simulink model "Simulink_serial_example"  (Simulink 10.0)
settings: Solver=FixedStepDiscrete  StartTime=0.0  StopTime=1056  RelTol=1e-3  EnableMultiTasking=on
undefined symbols (not defined in the file): D, fdesignblkfcn, gcbh
libraries: dspsigops x42, instrumentlib x1, dspsigattribs x1
settings Model: Creator=skolak  LastModifiedBy=bhisma
settings DataIOCC: LimitDataPoints=on  SignalLoggingSaveFormat=ModelDataLogs
settings OptimizationCC: InitFltsAndDblsToZero=on
settings DebuggingCC: SaveWithParameterizedLinksMsg=none  SignalResolutionControl=TryResolveAllWithWarning  SolverPrmCheckMsg=warning  MultiTaskDSMMsg=warning  MultiTaskCondExecSysMsg=none  FcnCallInpInsideContextMsg=warning
settings SFSimCC: SimUseLocalCustomCode=on  CustomCodeUndefinedFunction=FilterOut
settings RTWCC: RTWUseLocalCustomCode=on
settings GRTTargetCC: TargetFcnLib=ansi_tfl_tmw.mat

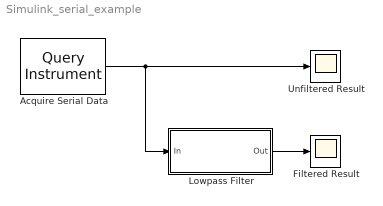
== system Simulink_serial_example ==
  Acquire Serial Data : instrumentlib/Query Instrument  sampleTime=1  isWorkspaceObject=off  timeout=10  inputBufferSize=10000  protocol=Serial  serialPort=COM1  baudRate=9600  gpibVendor=Advantech  boardIndex=0  primaryAddress=1  secondaryAddress=0  visaVendor=Agilent  visaSerialPort=0  chassisIndex=0  logicalAddress=0  tcpRemoteHost='127.0.0.1'  tcpRemotePort=4500  udpRemoteHost='127.0.0.1'  udpRemotePort=9090  visaTCPBoardIndex=0  visaTCPRemoteHost='127.0.0.1'  usbBoardIndex=0  usbManufID=0  usbModelCode=0  usbSerialNumber=0  initAction=Send ASCII Commands  initCommand='DATA:SOURCE CH1'  initFunction=get  queryCommand='curve?'  responseFormat=Binary  asciiFormatting='%d'  precision=16-bit integer  byteOrder=Little endian  valuesToRead=1056  removeBytes=on  afterOutputAction=Repeat query for new data  enableFrames=off  frameSize=1
      settings: SourceProductName=Instrument Control Toolbox  SourceProductBaseCode=IC
  Filtered Result : Scope
  Lowpass Filter : Subsystem  DialogController=fdesignblkfcn  DialogControllerArgs=DataTag1  InitFcn=fdesignblkfcn(gcbh, {'InitFcn'});  mask(Lowpass Filter){}
      mask help: Design a lowpass filter
      settings: CopyFcn=fdesignblkfcn(gcbh, {'CopyFcn'});
      mask Help: helpview(mapfilelocation('dspblks'), 'dsplowpassfilter')
      mask Display: disp('Lowpass')
  Unfiltered Result : Scope
  wires:
  Lowpass Filter/1(Out) -> Filtered Result/1
  Acquire Serial Data/1 -> Lowpass Filter/1(In), Unfiltered Result/1

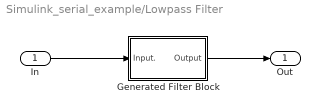
== system Simulink_serial_example/Lowpass Filter ==
  In : Inport
  Generated Filter Block : Subsystem  Tag=FilterWizardSubSystem
      settings: ErrorFcn=dspFilterRealizedInBasicElemsAlgLoopErrFcnCallback
  Out : Outport
  wires:
  In/1 -> Generated Filter Block/1(Input.)
  Generated Filter Block/1(Output) -> Out/1

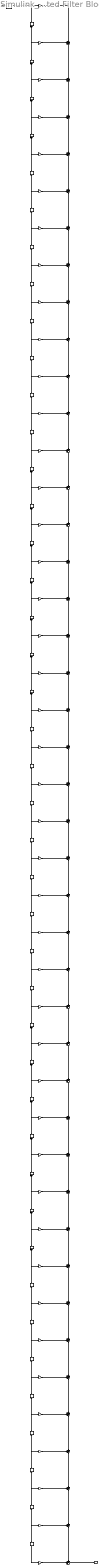
== system Simulink_serial_example/Lowpass Filter/Generated Filter Block ==
  Input. : Inport
  BodyDelay{2..43} (42 alike) : dspsigops/Delay  dly_unit=Samples  delay=1  ic_detail=off  dif_ic_for_ch=off  dif_ic_for_dly=off  ic=0  reset_popup=None
      settings: SourceProductName=DSP System Toolbox  SourceProductBaseCode=DS
  BodyLSum{2..43} (42 alike) : Sum  Inputs=++|  RndMeth=Nearest  SaturateOnIntegerOverflow=on  InputSameDT=on
  Input : dspsigattribs/Check Signal Attributes  SystemSampleTime=-1  SigAttribCheckMethod=Matches attributes exactly  Complexity=Ignore  Frame=Ignore  DimsCheckMethod=Ignore  Dimensions=1-D  DatatypeCheckMethod=Is not...  DatatypeGeneral=Floating-point  DtypeFloatSpecific=Any floating-point  DtypeFixedSpecific=Any fixed-point  DtypeIntSpecific=Any integer  SampleMode=Ignore
      settings: SourceProductName=DSP System Toolbox  SourceProductBaseCode=DS
  b(1) : Gain  Gain=-0.0024184515821339815  SaturateOnIntegerOverflow=on
  b(10) : Gain  Gain=-0.010109941080713171  SaturateOnIntegerOverflow=on
  b(11) : Gain  Gain=-0.018276710028363563  SaturateOnIntegerOverflow=on
  b(12) : Gain  Gain=0.011417030384770118  SaturateOnIntegerOverflow=on
  b(13) : Gain  Gain=0.026158313267711154  SaturateOnIntegerOverflow=on
  b(14) : Gain  Gain=-0.01249452054902888  SaturateOnIntegerOverflow=on
  b(15) : Gain  Gain=-0.037985890726300542  SaturateOnIntegerOverflow=on
  b(16) : Gain  Gain=0.013398022406508189  SaturateOnIntegerOverflow=on
  b(17) : Gain  Gain=0.058143561333869977  SaturateOnIntegerOverflow=on
  b(18) : Gain  Gain=-0.014068918704128731  SaturateOnIntegerOverflow=on
  b(19) : Gain  Gain=-0.10272737868066549  SaturateOnIntegerOverflow=on
  b(2) : Gain  Gain=-0.0020659659418839509  SaturateOnIntegerOverflow=on
  b(20) : Gain  Gain=0.014476257883398099  SaturateOnIntegerOverflow=on
  b(21) : Gain  Gain=0.31717292271198066  SaturateOnIntegerOverflow=on
  b(22) : Gain  Gain=0.48538538772192297  SaturateOnIntegerOverflow=on
  b(23) : Gain  Gain=0.31717292271198066  SaturateOnIntegerOverflow=on
  b(24) : Gain  Gain=0.014476257883398099  SaturateOnIntegerOverflow=on
  b(25) : Gain  Gain=-0.10272737868066549  SaturateOnIntegerOverflow=on
  b(26) : Gain  Gain=-0.014068918704128731  SaturateOnIntegerOverflow=on
  b(27) : Gain  Gain=0.058143561333869977  SaturateOnIntegerOverflow=on
  b(28) : Gain  Gain=0.013398022406508189  SaturateOnIntegerOverflow=on
  b(29) : Gain  Gain=-0.037985890726300542  SaturateOnIntegerOverflow=on
  b(3) : Gain  Gain=0.0067960727631209738  SaturateOnIntegerOverflow=on
  b(30) : Gain  Gain=-0.01249452054902888  SaturateOnIntegerOverflow=on
  b(31) : Gain  Gain=0.026158313267711154  SaturateOnIntegerOverflow=on
  b(32) : Gain  Gain=0.011417030384770118  SaturateOnIntegerOverflow=on
  b(33) : Gain  Gain=-0.018276710028363563  SaturateOnIntegerOverflow=on
  b(34) : Gain  Gain=-0.010109941080713171  SaturateOnIntegerOverflow=on
  b(35) : Gain  Gain=0.013006159969671948  SaturateOnIntegerOverflow=on
  b(36) : Gain  Gain=0.009274892431970062  SaturateOnIntegerOverflow=on
  b(37) : Gain  Gain=-0.0084078268149707022  SaturateOnIntegerOverflow=on
  b(38) : Gain  Gain=-0.0062562536117661332  SaturateOnIntegerOverflow=on
  b(39) : Gain  Gain=0.011103324338448677  SaturateOnIntegerOverflow=on
  b(4) : Gain  Gain=0.016745537375577622  SaturateOnIntegerOverflow=on
  b(40) : Gain  Gain=0.016745537375577622  SaturateOnIntegerOverflow=on
  b(41) : Gain  Gain=0.0067960727631209738  SaturateOnIntegerOverflow=on
  b(42) : Gain  Gain=-0.0020659659418839509  SaturateOnIntegerOverflow=on
  b(43) : Gain  Gain=-0.0024184515821339815  SaturateOnIntegerOverflow=on
  b(5) : Gain  Gain=0.011103324338448677  SaturateOnIntegerOverflow=on
  b(6) : Gain  Gain=-0.0062562536117661332  SaturateOnIntegerOverflow=on
  b(7) : Gain  Gain=-0.0084078268149707022  SaturateOnIntegerOverflow=on
  b(8) : Gain  Gain=0.009274892431970062  SaturateOnIntegerOverflow=on
  b(9) : Gain  Gain=0.013006159969671948  SaturateOnIntegerOverflow=on
  Output : Outport
  wires:
  Input./1 -> Input/1
  Input/1 -> b(1)/1, BodyDelay2/1
  b(1)/1 -> BodyLSum2/2
  BodyDelay2/1 -> b(2)/1, BodyDelay3/1
  b(2)/1 -> BodyLSum2/1
  BodyLSum2/1 -> BodyLSum3/2
  BodyDelay3/1 -> b(3)/1, BodyDelay4/1
  b(3)/1 -> BodyLSum3/1
  BodyLSum3/1 -> BodyLSum4/2
  BodyDelay4/1 -> b(4)/1, BodyDelay5/1
  b(4)/1 -> BodyLSum4/1
  BodyLSum4/1 -> BodyLSum5/2
  BodyDelay5/1 -> b(5)/1, BodyDelay6/1
  b(5)/1 -> BodyLSum5/1
  BodyLSum5/1 -> BodyLSum6/2
  BodyDelay6/1 -> b(6)/1, BodyDelay7/1
  b(6)/1 -> BodyLSum6/1
  BodyLSum6/1 -> BodyLSum7/2
  BodyDelay7/1 -> b(7)/1, BodyDelay8/1
  b(7)/1 -> BodyLSum7/1
  BodyLSum7/1 -> BodyLSum8/2
  BodyDelay8/1 -> b(8)/1, BodyDelay9/1
  b(8)/1 -> BodyLSum8/1
  BodyLSum8/1 -> BodyLSum9/2
  BodyDelay9/1 -> b(9)/1, BodyDelay10/1
  b(9)/1 -> BodyLSum9/1
  BodyLSum9/1 -> BodyLSum10/2
  BodyDelay10/1 -> b(10)/1, BodyDelay11/1
  b(10)/1 -> BodyLSum10/1
  BodyLSum10/1 -> BodyLSum11/2
  BodyDelay11/1 -> b(11)/1, BodyDelay12/1
  b(11)/1 -> BodyLSum11/1
  BodyLSum11/1 -> BodyLSum12/2
  BodyDelay12/1 -> b(12)/1, BodyDelay13/1
  b(12)/1 -> BodyLSum12/1
  BodyLSum12/1 -> BodyLSum13/2
  BodyDelay13/1 -> b(13)/1, BodyDelay14/1
  b(13)/1 -> BodyLSum13/1
  BodyLSum13/1 -> BodyLSum14/2
  BodyDelay14/1 -> b(14)/1, BodyDelay15/1
  b(14)/1 -> BodyLSum14/1
  BodyLSum14/1 -> BodyLSum15/2
  BodyDelay15/1 -> b(15)/1, BodyDelay16/1
  b(15)/1 -> BodyLSum15/1
  BodyLSum15/1 -> BodyLSum16/2
  BodyDelay16/1 -> b(16)/1, BodyDelay17/1
  b(16)/1 -> BodyLSum16/1
  BodyLSum16/1 -> BodyLSum17/2
  BodyDelay17/1 -> b(17)/1, BodyDelay18/1
  b(17)/1 -> BodyLSum17/1
  BodyLSum17/1 -> BodyLSum18/2
  BodyDelay18/1 -> b(18)/1, BodyDelay19/1
  b(18)/1 -> BodyLSum18/1
  BodyLSum18/1 -> BodyLSum19/2
  BodyDelay19/1 -> b(19)/1, BodyDelay20/1
  b(19)/1 -> BodyLSum19/1
  BodyLSum19/1 -> BodyLSum20/2
  BodyDelay20/1 -> b(20)/1, BodyDelay21/1
  b(20)/1 -> BodyLSum20/1
  BodyLSum20/1 -> BodyLSum21/2
  BodyDelay21/1 -> b(21)/1, BodyDelay22/1
  b(21)/1 -> BodyLSum21/1
  BodyLSum21/1 -> BodyLSum22/2
  BodyDelay22/1 -> b(22)/1, BodyDelay23/1
  b(22)/1 -> BodyLSum22/1
  BodyLSum22/1 -> BodyLSum23/2
  BodyDelay23/1 -> b(23)/1, BodyDelay24/1
  b(23)/1 -> BodyLSum23/1
  BodyLSum23/1 -> BodyLSum24/2
  BodyDelay24/1 -> b(24)/1, BodyDelay25/1
  b(24)/1 -> BodyLSum24/1
  BodyLSum24/1 -> BodyLSum25/2
  BodyDelay25/1 -> b(25)/1, BodyDelay26/1
  b(25)/1 -> BodyLSum25/1
  BodyLSum25/1 -> BodyLSum26/2
  BodyDelay26/1 -> b(26)/1, BodyDelay27/1
  b(26)/1 -> BodyLSum26/1
  BodyLSum26/1 -> BodyLSum27/2
  BodyDelay27/1 -> b(27)/1, BodyDelay28/1
  b(27)/1 -> BodyLSum27/1
  BodyLSum27/1 -> BodyLSum28/2
  BodyDelay28/1 -> b(28)/1, BodyDelay29/1
  b(28)/1 -> BodyLSum28/1
  BodyLSum28/1 -> BodyLSum29/2
  BodyDelay29/1 -> b(29)/1, BodyDelay30/1
  b(29)/1 -> BodyLSum29/1
  BodyLSum29/1 -> BodyLSum30/2
  BodyDelay30/1 -> b(30)/1, BodyDelay31/1
  b(30)/1 -> BodyLSum30/1
  BodyLSum30/1 -> BodyLSum31/2
  BodyDelay31/1 -> b(31)/1, BodyDelay32/1
  b(31)/1 -> BodyLSum31/1
  BodyLSum31/1 -> BodyLSum32/2
  BodyDelay32/1 -> b(32)/1, BodyDelay33/1
  b(32)/1 -> BodyLSum32/1
  BodyLSum32/1 -> BodyLSum33/2
  BodyDelay33/1 -> b(33)/1, BodyDelay34/1
  b(33)/1 -> BodyLSum33/1
  BodyLSum33/1 -> BodyLSum34/2
  BodyDelay34/1 -> b(34)/1, BodyDelay35/1
  b(34)/1 -> BodyLSum34/1
  BodyLSum34/1 -> BodyLSum35/2
  BodyDelay35/1 -> b(35)/1, BodyDelay36/1
  b(35)/1 -> BodyLSum35/1
  BodyLSum35/1 -> BodyLSum36/2
  BodyDelay36/1 -> b(36)/1, BodyDelay37/1
  b(36)/1 -> BodyLSum36/1
  BodyLSum36/1 -> BodyLSum37/2
  BodyDelay37/1 -> b(37)/1, BodyDelay38/1
  b(37)/1 -> BodyLSum37/1
  BodyLSum37/1 -> BodyLSum38/2
  BodyDelay38/1 -> b(38)/1, BodyDelay39/1
  b(38)/1 -> BodyLSum38/1
  BodyLSum38/1 -> BodyLSum39/2
  BodyDelay39/1 -> b(39)/1, BodyDelay40/1
  b(39)/1 -> BodyLSum39/1
  BodyLSum39/1 -> BodyLSum40/2
  BodyDelay40/1 -> b(40)/1, BodyDelay41/1
  b(40)/1 -> BodyLSum40/1
  BodyLSum40/1 -> BodyLSum41/2
  BodyDelay41/1 -> b(41)/1, BodyDelay42/1
  b(41)/1 -> BodyLSum41/1
  BodyLSum41/1 -> BodyLSum42/2
  BodyDelay42/1 -> b(42)/1, BodyDelay43/1
  b(42)/1 -> BodyLSum42/1
  BodyLSum42/1 -> BodyLSum43/1
  BodyDelay43/1 -> b(43)/1
  b(43)/1 -> BodyLSum43/2
  BodyLSum43/1 -> Output/1
